simulink model "SMA_displacementIn_PC2"  (R2018a)
settings: Solver=ode15s  StartTime=0.0  StopTime=100  RelTol=1e-8  AbsTol=1e-8  EnableMultiTasking=on
values from neighbouring files (symbols this model uses):
  param_N = 10    [plot_task_1.m]
undefined symbols (not defined in the file or in its folder): param_J, param_K, param_y0, params_PC2
libraries: simulink x1
settings Model: Creator=Gianluca  LastModifiedBy=tim
settings SolverCC: AutoScaleAbsTol=off
settings DataIOCC: LimitDataPoints=on  SaveFormat=Array
settings OptimizationCC: LifeSpan=inf
settings DebuggingCC: UnderspecifiedInitializationDetection=Classic  MergeDetectMultiDrivingBlocksExec=none  SolverPrmCheckMsg=warning  StateNameClashWarn=warning  SFUnexpectedBacktrackingDiag=warning  SFNoUnconditionalDefaultTransitionDiag=warning  SFExecutionAtInitializationDiag=none
settings HardwareCC: ProdBitPerPointer=32  ProdBitPerSizeT=32  ProdBitPerPtrDiffT=32  ProdLargestAtomicFloat=None  ProdIntDivRoundTo=Undefined  ProdEndianess=Unspecified  ProdWordSize=32  ProdHWDeviceType=32-bit Generic
settings ModelReferenceCC: PropagateSignalLabelsOutOfModel=off
settings CodeAppCC: StateflowObjectComments=on
settings GRTTargetCC: TargetLangStandard=C89/C90 (ANSI)  GeneratePreprocessorConditionals=Disable all
settings ConfigComp: CovMetricSettings=dw  CovHtmlReporting=on  CovSaveCumulativeToWorkspaceVar=on  CovSaveSingleToWorkspaceVar=on  CovExternalEMLEnable=off

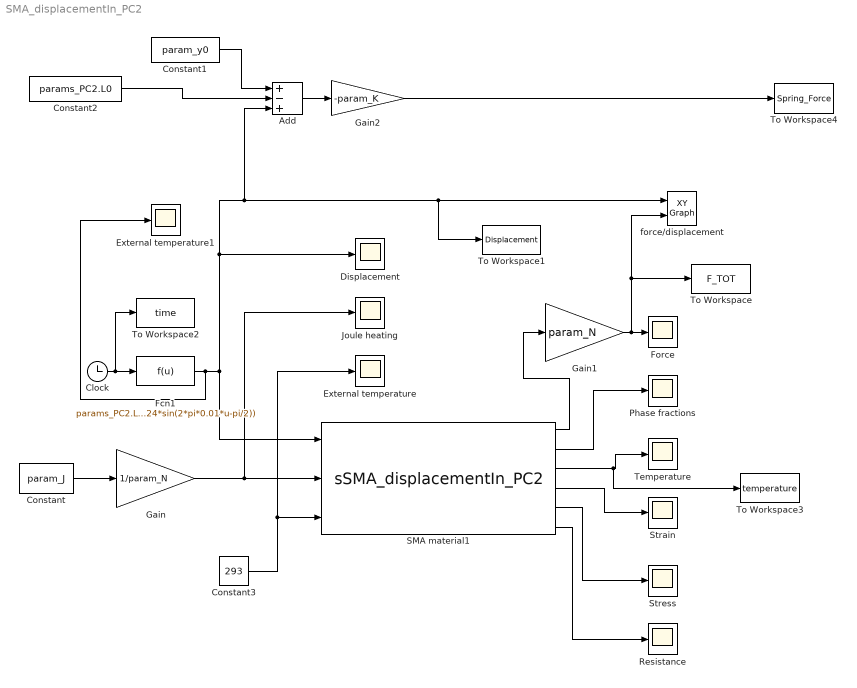
== system SMA_displacementIn_PC2 ==
  Add : Sum  Inputs=+-+
  Clock : Clock
  Constant : Constant  Value=param_J
  Constant1 : Constant  Value=param_y0
  Constant2 : Constant  Value=params_PC2.L0
  Constant3 : Constant  Value=293
  Displacement : Scope
  External temperature : Scope
  External temperature1 : Scope
  Fcn1 : Fcn  Expr=params_PC2.L0*(1.024 + 0.024*sin(2*pi*0.01*u-pi/2))
  Force : Scope
  Gain : Gain  Gain=1/param_N
  Gain1 : Gain  Gain=param_N
  Gain2 : Gain  Gain=-param_K
  Joule heating : Scope
  Phase fractions : Scope
  Resistance : Scope
  SMA material1 : M-S-Function  FunctionName=sSMA_displacementIn_PC2  Parameters=params_PC2, initConds_PC2
      mask Display:
      | color('black');
      | patch(3*[-1 1 1 -1],1.1*[-1 -1 1 1],[1 1 1]);
      | patch([-1.6 -0.8],[-0.9 0.3],[0 0 0]);
      | patch([-0.8 1.2],[0.3 0.3],[0 0 0]);
      | patch([1.6 0.8],[0.9 -0.3],[0 0 0]);
      | patch([0.8 -1.2],[-0.3 -0.3],[0 0 0]);
      | disp('SMA');
      | 
      | color('blue');
      | port_label('input', 1, 'y [m]','texmode','on');
      | port_label('input', 2, 'J [W]','texmode','on');
      | port_label('input', 3, 'T_E [K]','texmode','on');
      | 
      | color('red');
      | port_label('output', 1, 'F [N]','texmode','on');
      | port_label('output', 2, 'x_+, x_-, x_A [-]','texmode','on');
      | port_label('output', 3, 'T [K]','texmode','on');
      | port_label('output', 4, '\epsilon [-]','texmode','on');
      | port_label('output', 5, '\sigma [Pa]','texmode','on');
      | port_label('output', 6, 'R [\Omega]','texmode','on');
  Strain : Scope
  Stress : Scope
  Temperature : Scope
  To Workspace : ToWorkspace  VariableName=F_TOT  SampleTime=-1
  To Workspace1 : ToWorkspace  VariableName=Displacement  SampleTime=-1
  To Workspace2 : ToWorkspace  VariableName=time  SampleTime=-1
  To Workspace3 : ToWorkspace  VariableName=temperature  SampleTime=-1
  To Workspace4 : ToWorkspace  VariableName=Spring_Force  SampleTime=-1
  force/displacement : simulink/Sinks/XY Graph  xmin=0.1  xmax=0.106  ymin=0  ymax=2.5  st=-1
  wires:
  Gain/1 -> Joule heating/1, SMA material1/2
  Constant3/1 -> SMA material1/3, External temperature/1
  SMA material1/2 -> Phase fractions/1
  SMA material1/3 -> To Workspace3/1, Temperature/1
  SMA material1/4 -> Strain/1
  SMA material1/5 -> Stress/1
  SMA material1/6 -> Resistance/1
  Clock/1 -> To Workspace2/1, Fcn1/1
  Fcn1/1 -> External temperature1/1, SMA material1/1, Add/3, To Workspace1/1, force/displacement/1, Displacement/1
  Constant/1 -> Gain/1
  Gain1/1 -> To Workspace/1, force/displacement/2, Force/1
  SMA material1/1 -> Gain1/1
  Constant2/1 -> Add/2
  Constant1/1 -> Add/1
  Add/1 -> Gain2/1
  Gain2/1 -> To Workspace4/1
